simulink model "TALLER1"  (R2025a)
settings: Solver=VariableStepAuto  StartTime=0.0  StopTime=10.0  RelTol=1e-3

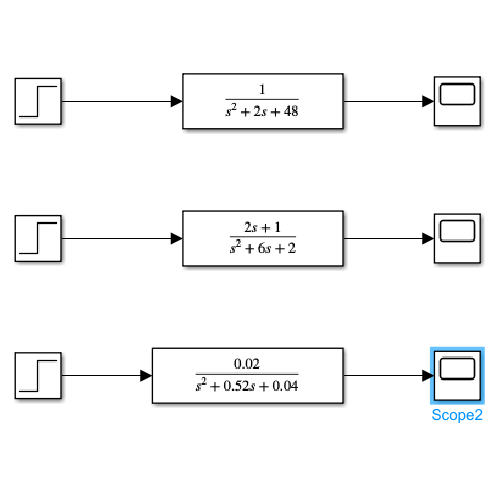
[thumbnail: Simulink's stored preview of the top-level diagram]
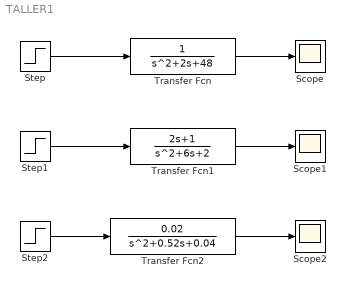
== system TALLER1 ==
  Scope : Scope
  Scope1 : Scope
  Scope2 : Scope
  Step : Step  Time=0  SampleTime=0
  Step1 : Step  Time=0  SampleTime=0
  Step2 : Step  Time=0  SampleTime=0
  Transfer Fcn : TransferFcn  Denominator=[1 2 48]
  Transfer Fcn1 : TransferFcn  Numerator=[2 1]  Denominator=[1 6 2]
  Transfer Fcn2 : TransferFcn  Numerator=[0.02]  Denominator=[1 0.52 0.04]
  wires:
  Step/1 -> Transfer Fcn/1
  Transfer Fcn/1 -> Scope/1
  Transfer Fcn1/1 -> Scope1/1
  Step1/1 -> Transfer Fcn1/1
  Transfer Fcn2/1 -> Scope2/1
  Step2/1 -> Transfer Fcn2/1
